simulink library "Orientation_Library"  (Simulink 8.0)
settings: Solver=ode1  StartTime=0.0  StopTime=inf  FixedStep=0.002  RelTol=1e-3
undefined symbols (not defined in the file or in its folder): qc_get_step_size
libraries: Orientation_Library x28, quarc_library x2, simulink x1
settings Model: Creator=glai  LastModifiedBy=glai  ExtModeTrigDuration=5000

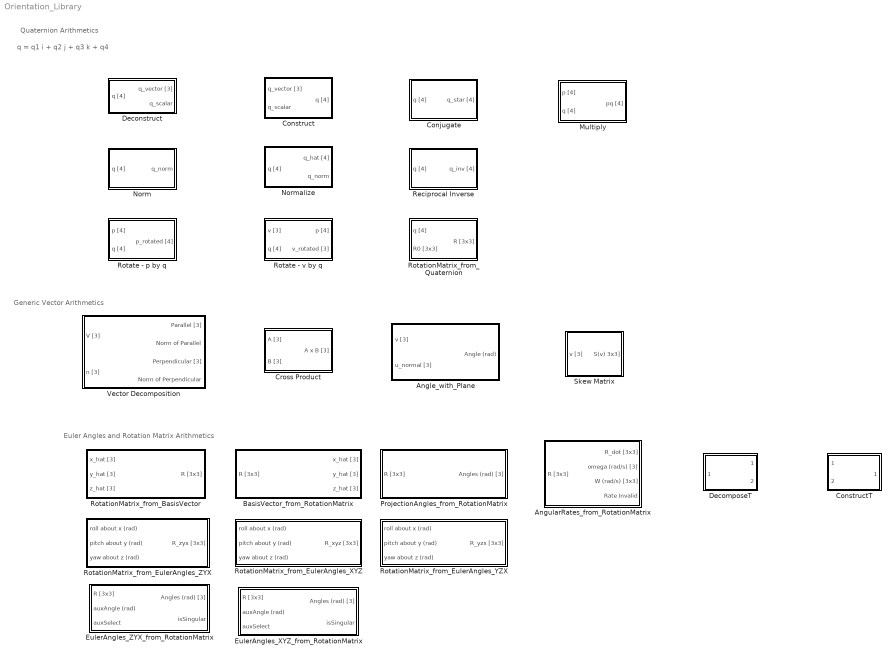
== system Orientation_Library ==
  note: Quaternion Arithmetics
  note: q = q1 i + q2 j + q3 k + q4
  note: Generic Vector Arithmetics
  note: Euler Angles and Rotation Matrix Arithmetics
  Angle_with_Plane : Subsystem
  AngularRates_from_RotationMatrix : Subsystem
  BasisVector_from_RotationMatrix : Subsystem
  Conjugate : Subsystem
  Construct : Subsystem
  ConstructT : Subsystem
  Cross Product : Subsystem
  DecomposeT : Subsystem
  Deconstruct : Subsystem
  EulerAngles_XYZ_from_RotationMatrix : Subsystem
  EulerAngles_ZYX_from_RotationMatrix : Subsystem
  Multiply : Subsystem
  Norm : Subsystem
  Normalize : Subsystem
  ProjectionAngles_from_RotationMatrix : Subsystem
  Reciprocal Inverse : Subsystem
  Rotate - p by q : Subsystem
  Rotate - v by q : Subsystem
  RotationMatrix_from_BasisVector : Subsystem
  RotationMatrix_from_EulerAngles_XYZ : Subsystem
  RotationMatrix_from_EulerAngles_YZX : Subsystem
  RotationMatrix_from_EulerAngles_ZYX : Subsystem
  RotationMatrix_from_Quaternion : Subsystem
  Skew Matrix : Subsystem
  Vector Decomposition : Subsystem

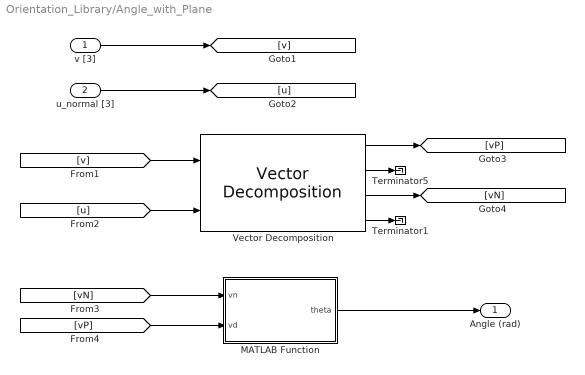
== system Orientation_Library/Angle_with_Plane ==
  v [3] : Inport
  u_normal [3] : Inport  Port=2
  MATLAB Function : MATLAB Function  TreatAsAtomicUnit=on
      settings: PermitHierarchicalResolution=ParametersOnly
  Terminator1 : Terminator
  Terminator5 : Terminator
  Vector Decomposition : Orientation_Library/Vector Decomposition
  Angle (rad) : Outport
  wires:
  v [3]/1 -> [v]
  u_normal [3]/1 -> [u]
  [v] -> Vector Decomposition/1
  [u] -> Vector Decomposition/2
  Vector Decomposition/1 -> [vP]
  Vector Decomposition/2 -> Terminator5/1
  Vector Decomposition/3 -> [vN]
  Vector Decomposition/4 -> Terminator1/1
  MATLAB Function/1(theta) -> Angle (rad)/1
  [vN] -> MATLAB Function/1(vn)
  [vP] -> MATLAB Function/2(vd)

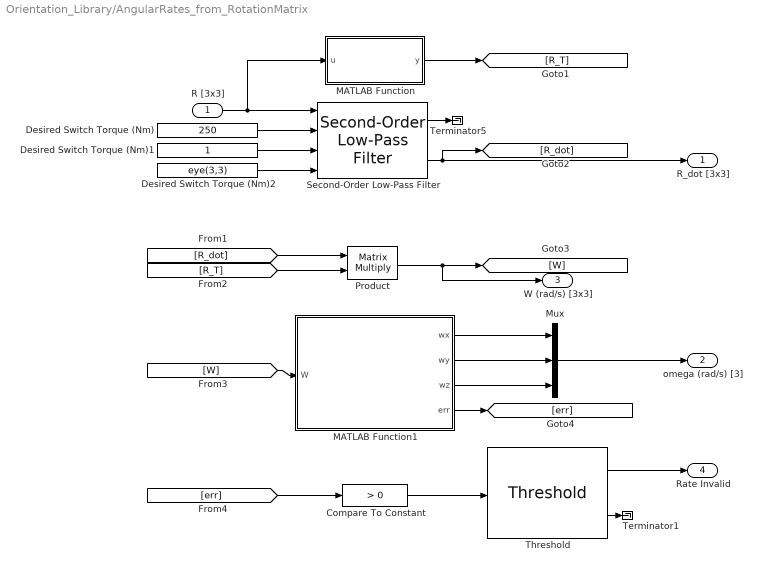
== system Orientation_Library/AngularRates_from_RotationMatrix ==
  R [3x3] : Inport
  Compare To Constant : simulink/Logic and Bit Operations/Compare To Constant  relop=>  const=0  OutDataTypeStr=uint8
  Desired Switch Torque (Nm) : Constant  Value=250
  Desired Switch Torque (Nm)1 : Constant
  Desired Switch Torque (Nm)2 : Constant  Value=eye(3,3)
  MATLAB Function : MATLAB Function  TreatAsAtomicUnit=on
      settings: PermitHierarchicalResolution=ParametersOnly
  MATLAB Function1 : MATLAB Function  TreatAsAtomicUnit=on
      settings: PermitHierarchicalResolution=ParametersOnly
  Mux : Mux  Inputs=3
  Product : Product  Multiplication=Matrix(*)  RndMeth=Zero
  Second-Order Low-Pass Filter : quarc_library/Continuous/Second-Order Low-Pass Filter  params_source=External (input ports)  input_width=1  input_zeta=1  input_init=0
  Terminator1 : Terminator
  Terminator5 : Terminator
  Threshold : quarc_library/Discontinuities/Threshold  operator=>  param_src=Specify via dialog  threshold=0  duration=qc_get_step_size*5000
  R_dot [3x3] : Outport
  omega (rad/s) [3] : Outport  Port=2
  W (rad/s) [3x3] : Outport  Port=3
  Rate Invalid : Outport  Port=4
  wires:
  Threshold/1 -> Rate Invalid/1
  Threshold/2 -> Terminator1/1
  Compare To Constant/1 -> Threshold/1
  Desired Switch Torque (Nm)2/1 -> Second-Order Low-Pass Filter/4
  Desired Switch Torque (Nm)1/1 -> Second-Order Low-Pass Filter/3
  Desired Switch Torque (Nm)/1 -> Second-Order Low-Pass Filter/2
  [err] -> Compare To Constant/1
  Mux/1 -> omega (rad/s) [3]/1
  MATLAB Function1/4(err) -> [err]
  MATLAB Function1/3(wz) -> Mux/3
  MATLAB Function1/2(wy) -> Mux/2
  MATLAB Function1/1(wx) -> Mux/1
  [W] -> MATLAB Function1/1(W)
  Product/1 -> W (rad/s) [3x3]/1, [W]
  [R_T] -> Product/2
  MATLAB Function/1(y) -> [R_T]
  [R_dot] -> Product/1
  Second-Order Low-Pass Filter/2 -> [R_dot], R_dot [3x3]/1
  Second-Order Low-Pass Filter/1 -> Terminator5/1
  R [3x3]/1 -> MATLAB Function/1(u), Second-Order Low-Pass Filter/1

== system Orientation_Library/BasisVector_from_RotationMatrix ==
  R [3x3] : Inport
  BasisVector_from_RotationMatrix : MATLAB Function  TreatAsAtomicUnit=on
      settings: PermitHierarchicalResolution=ParametersOnly
  x_hat [3] : Outport
  y_hat [3] : Outport  Port=2
  z_hat [3] : Outport  Port=3
  wires:
  R [3x3]/1 -> BasisVector_from_RotationMatrix/1(R)
  BasisVector_from_RotationMatrix/1(x_hat) -> x_hat [3]/1
  BasisVector_from_RotationMatrix/2(y_hat) -> y_hat [3]/1
  BasisVector_from_RotationMatrix/3(z_hat) -> z_hat [3]/1

== system Orientation_Library/Conjugate ==
  q [4] : Inport
  Demux : Demux  Outputs=[3 1]
  Gain : Gain  Gain=-1
  Mux : Mux  Inputs=[3 1]
  q_star [4] : Outport
  wires:
  Demux/1 -> Gain/1
  Gain/1 -> Mux/1
  Demux/2 -> Mux/2
  q [4]/1 -> Demux/1
  Mux/1 -> q_star [4]/1

== system Orientation_Library/Construct ==
  q_vector [3] : Inport
  q_scalar : Inport  Port=2
  Mux : Mux  Inputs=[3 1]
  q [4] : Outport
  wires:
  Mux/1 -> q [4]/1
  q_vector [3]/1 -> Mux/1
  q_scalar/1 -> Mux/2

== system Orientation_Library/ConstructT ==
  R [3x3] : Inport
  P (m) [3] : Inport  Port=2
  MATLAB Function3 : MATLAB Function  TreatAsAtomicUnit=on
      settings: PermitHierarchicalResolution=ParametersOnly
  T [4x4] : Outport
  wires:
  MATLAB Function3/1(T) -> T [4x4]/1
  P (m) [3]/1 -> MATLAB Function3/2(P)
  R [3x3]/1 -> MATLAB Function3/1(R)

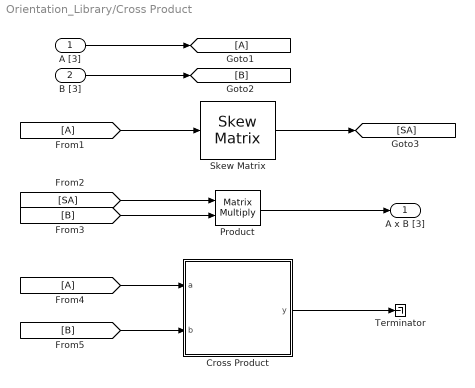
== system Orientation_Library/Cross Product ==
  A [3] : Inport
  B [3] : Inport  Port=2
  Cross Product : MATLAB Function  TreatAsAtomicUnit=on
      settings: PermitHierarchicalResolution=ParametersOnly
  Product : Product  Multiplication=Matrix(*)  RndMeth=Zero
  Skew Matrix : Orientation_Library/Skew Matrix
  Terminator : Terminator
  A x B [3] : Outport
  wires:
  B [3]/1 -> [B]
  A [3]/1 -> [A]
  [A] -> Skew Matrix/1
  Skew Matrix/1 -> [SA]
  [SA] -> Product/1
  [B] -> Product/2
  Product/1 -> A x B [3]/1
  [A] -> Cross Product/1(a)
  [B] -> Cross Product/2(b)
  Cross Product/1(y) -> Terminator/1

== system Orientation_Library/DecomposeT ==
  T [4x4] : Inport
  MATLAB Function1 : MATLAB Function  TreatAsAtomicUnit=on
      settings: PermitHierarchicalResolution=ParametersOnly
  R [3x3] : Outport
  P (m) [3] : Outport  Port=2
  wires:
  MATLAB Function1/2(P) -> P (m) [3]/1
  MATLAB Function1/1(R) -> R [3x3]/1
  T [4x4]/1 -> MATLAB Function1/1(T)

== system Orientation_Library/Deconstruct ==
  q [4] : Inport
  Demux : Demux  Outputs=[3 1]
  q_vector [3] : Outport
  q_scalar : Outport  Port=2
  wires:
  q [4]/1 -> Demux/1
  Demux/1 -> q_vector [3]/1
  Demux/2 -> q_scalar/1

== system Orientation_Library/EulerAngles_XYZ_from_RotationMatrix ==
  R [3x3] : Inport
  auxAngle (rad) : Inport  Port=2
  auxSelect : Inport  Port=3
  EulerAngles_xyz_from_RotationMatrix : MATLAB Function  TreatAsAtomicUnit=on
      settings: PermitHierarchicalResolution=ParametersOnly
  Angles (rad) [3] : Outport
  isSingular : Outport  Port=2
  wires:
  EulerAngles_xyz_from_RotationMatrix/1(Angles) -> Angles (rad) [3]/1
  EulerAngles_xyz_from_RotationMatrix/2(isSingular) -> isSingular/1
  R [3x3]/1 -> EulerAngles_xyz_from_RotationMatrix/1(R)
  auxAngle (rad)/1 -> EulerAngles_xyz_from_RotationMatrix/2(auxAngle)
  auxSelect/1 -> EulerAngles_xyz_from_RotationMatrix/3(auxSelect)

== system Orientation_Library/EulerAngles_ZYX_from_RotationMatrix ==
  R [3x3] : Inport
  auxAngle (rad) : Inport  Port=2
  auxSelect : Inport  Port=3
  EulerAngles_zyx_from_RotationMatrix : MATLAB Function  TreatAsAtomicUnit=on
      settings: PermitHierarchicalResolution=ParametersOnly
  Angles (rad) [3] : Outport
  isSingular : Outport  Port=2
  wires:
  EulerAngles_zyx_from_RotationMatrix/2(isSingular) -> isSingular/1
  EulerAngles_zyx_from_RotationMatrix/1(Angles) -> Angles (rad) [3]/1
  auxSelect/1 -> EulerAngles_zyx_from_RotationMatrix/3(auxSelect)
  auxAngle (rad)/1 -> EulerAngles_zyx_from_RotationMatrix/2(auxAngle)
  R [3x3]/1 -> EulerAngles_zyx_from_RotationMatrix/1(R)

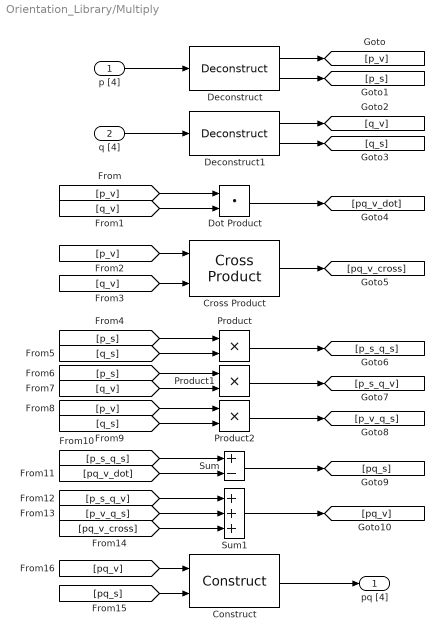
== system Orientation_Library/Multiply ==
  p [4] : Inport
  q [4] : Inport  Port=2
  Construct : Orientation_Library/Construct
  Cross Product : Orientation_Library/Cross Product
  Deconstruct : Orientation_Library/Deconstruct
  Deconstruct1 : Orientation_Library/Deconstruct
  Dot Product : DotProduct  InputSameDT=on  OutDataTypeStr=Inherit: Inherit via internal rule
  Product : Product  RndMeth=Zero
  Product1 : Product  RndMeth=Zero
  Product2 : Product  RndMeth=Zero
  Sum : Sum  Inputs=+-
  Sum1 : Sum  Inputs=+++
  pq [4] : Outport
  wires:
  p [4]/1 -> Deconstruct/1
  q [4]/1 -> Deconstruct1/1
  Deconstruct/1 -> [p_v]
  Deconstruct/2 -> [p_s]
  Deconstruct1/1 -> [q_v]
  Deconstruct1/2 -> [q_s]
  [p_v] -> Dot Product/1
  [q_v] -> Dot Product/2
  Dot Product/1 -> [pq_v_dot]
  [p_v] -> Cross Product/1
  [q_v] -> Cross Product/2
  Cross Product/1 -> [pq_v_cross]
  [p_s] -> Product/1
  [q_s] -> Product/2
  Product/1 -> [p_s_q_s]
  [p_s] -> Product1/1
  [q_v] -> Product1/2
  Product1/1 -> [p_s_q_v]
  [p_v] -> Product2/1
  [q_s] -> Product2/2
  Product2/1 -> [p_v_q_s]
  [p_s_q_s] -> Sum/1
  [pq_v_dot] -> Sum/2
  Sum/1 -> [pq_s]
  [p_s_q_v] -> Sum1/1
  [p_v_q_s] -> Sum1/2
  Sum1/1 -> [pq_v]
  [pq_v_cross] -> Sum1/3
  [pq_v] -> Construct/1
  [pq_s] -> Construct/2
  Construct/1 -> pq [4]/1

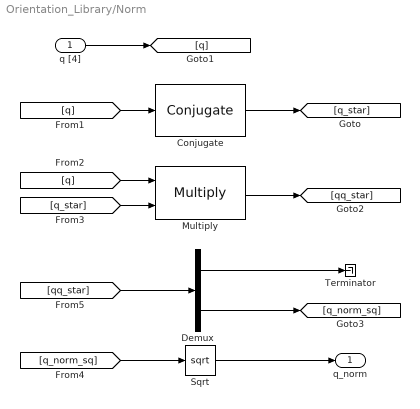
== system Orientation_Library/Norm ==
  q [4] : Inport
  Conjugate : Orientation_Library/Conjugate
  Demux : Demux  Outputs=[3 1]
  Multiply : Orientation_Library/Multiply
  Sqrt : Sqrt  SaturateOnIntegerOverflow=on
  Terminator : Terminator
  q_norm : Outport
  wires:
  Conjugate/1 -> [q_star]
  q [4]/1 -> [q]
  [q] -> Conjugate/1
  [q_norm_sq] -> Sqrt/1
  Sqrt/1 -> q_norm/1
  [q] -> Multiply/1
  [q_star] -> Multiply/2
  Multiply/1 -> [qq_star]
  [qq_star] -> Demux/1
  Demux/1 -> Terminator/1
  Demux/2 -> [q_norm_sq]

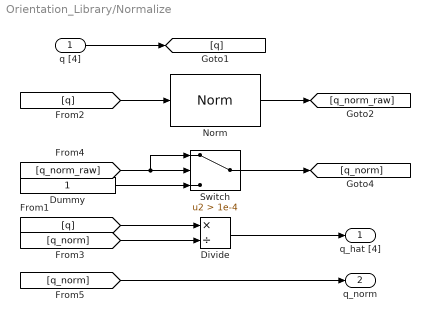
== system Orientation_Library/Normalize ==
  q [4] : Inport
  Divide : Product  Inputs=*/
  Dummy : Constant
  Norm : Orientation_Library/Norm
  Switch : Switch  Criteria=u2 > Threshold  Threshold=1e-4
  q_hat [4] : Outport
  q_norm : Outport  Port=2
  wires:
  q [4]/1 -> [q]
  Norm/1 -> [q_norm_raw]
  [q] -> Norm/1
  [q] -> Divide/1
  [q_norm] -> Divide/2
  [q_norm_raw] -> Switch/1, Switch/2
  Dummy/1 -> Switch/3
  Switch/1 -> [q_norm]
  Divide/1 -> q_hat [4]/1
  [q_norm] -> q_norm/1

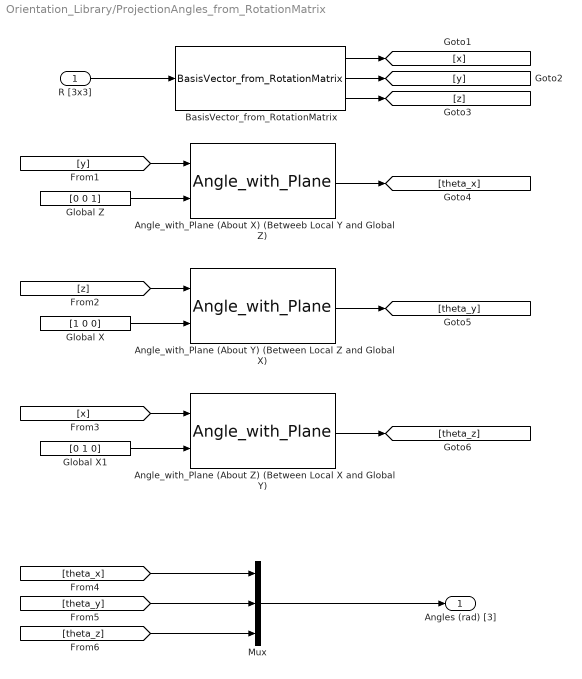
== system Orientation_Library/ProjectionAngles_from_RotationMatrix ==
  R [3x3] : Inport
  "Angle_with_Plane (About X) (Betweeb Local Y and Global Z) " : Orientation_Library/Angle_with_Plane
  Angle_with_Plane (About Y) (Between Local Z and Global X) : Orientation_Library/Angle_with_Plane
  Angle_with_Plane (About Z) (Between Local X and Global Y) : Orientation_Library/Angle_with_Plane
  BasisVector_from_RotationMatrix : Orientation_Library/BasisVector_from_RotationMatrix
  Global X : Constant  Value=[1 0 0]
  Global X1 : Constant  Value=[0 1 0]
  Global Z : Constant  Value=[0 0 1]
  Mux : Mux  Inputs=3
  Angles (rad) [3] : Outport
  wires:
  R [3x3]/1 -> BasisVector_from_RotationMatrix/1
  [y] -> "Angle_with_Plane (About X) (Betweeb Local Y and Global Z) "/1
  Global Z/1 -> "Angle_with_Plane (About X) (Betweeb Local Y and Global Z) "/2
  "Angle_with_Plane (About X) (Betweeb Local Y and Global Z) "/1 -> [theta_x]
  [z] -> Angle_with_Plane (About Y) (Between Local Z and Global X)/1
  Global X/1 -> Angle_with_Plane (About Y) (Between Local Z and Global X)/2
  Angle_with_Plane (About Y) (Between Local Z and Global X)/1 -> [theta_y]
  [x] -> Angle_with_Plane (About Z) (Between Local X and Global Y)/1
  Global X1/1 -> Angle_with_Plane (About Z) (Between Local X and Global Y)/2
  Angle_with_Plane (About Z) (Between Local X and Global Y)/1 -> [theta_z]
  Mux/1 -> Angles (rad) [3]/1
  [theta_x] -> Mux/1
  [theta_y] -> Mux/2
  [theta_z] -> Mux/3
  BasisVector_from_RotationMatrix/1 -> [x]
  BasisVector_from_RotationMatrix/2 -> [y]
  BasisVector_from_RotationMatrix/3 -> [z]

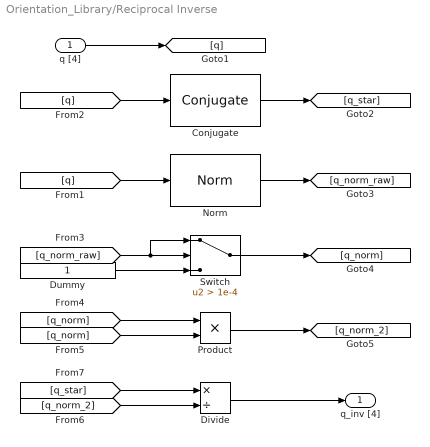
== system Orientation_Library/Reciprocal Inverse ==
  q [4] : Inport
  Conjugate : Orientation_Library/Conjugate
  Divide : Product  Inputs=*/
  Dummy : Constant
  Norm : Orientation_Library/Norm
  Product : Product  RndMeth=Zero
  Switch : Switch  Criteria=u2 > Threshold  Threshold=1e-4
  q_inv [4] : Outport
  wires:
  q [4]/1 -> [q]
  [q] -> Conjugate/1
  Conjugate/1 -> [q_star]
  [q] -> Norm/1
  Norm/1 -> [q_norm_raw]
  [q_norm_raw] -> Switch/1, Switch/2
  Dummy/1 -> Switch/3
  Switch/1 -> [q_norm]
  [q_norm] -> Product/1
  [q_norm] -> Product/2
  Product/1 -> [q_norm_2]
  [q_star] -> Divide/1
  [q_norm_2] -> Divide/2
  Divide/1 -> q_inv [4]/1

== system Orientation_Library/Rotate - p by q ==
  p [4] : Inport
  q [4] : Inport  Port=2
  Multiply : Orientation_Library/Multiply
  Multiply1 : Orientation_Library/Multiply
  Reciprocal Inverse : Orientation_Library/Reciprocal Inverse
  p_rotated [4] : Outport
  wires:
  Multiply/1 -> [qp]
  [p] -> Multiply/2
  [q] -> Multiply/1
  [q] -> Reciprocal Inverse/1
  p [4]/1 -> [p]
  Reciprocal Inverse/1 -> [q_inv]
  q [4]/1 -> [q]
  [qp] -> Multiply1/1
  [q_inv] -> Multiply1/2
  Multiply1/1 -> p_rotated [4]/1

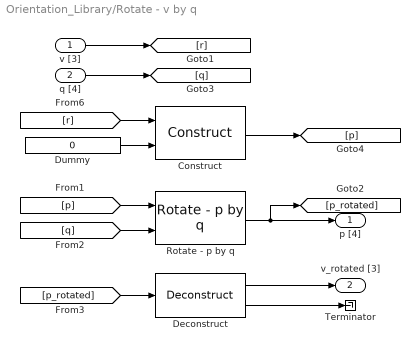
== system Orientation_Library/Rotate - v by q ==
  v [3] : Inport
  q [4] : Inport  Port=2
  Construct : Orientation_Library/Construct
  Deconstruct : Orientation_Library/Deconstruct
  Dummy : Constant  Value=0
  Rotate - p by q : Orientation_Library/Rotate - p by q
  Terminator : Terminator
  p [4] : Outport
  v_rotated [3] : Outport  Port=2
  wires:
  q [4]/1 -> [q]
  v [3]/1 -> [r]
  [r] -> Construct/1
  Dummy/1 -> Construct/2
  Construct/1 -> [p]
  [p] -> Rotate - p by q/1
  [q] -> Rotate - p by q/2
  Rotate - p by q/1 -> p [4]/1, [p_rotated]
  Deconstruct/1 -> v_rotated [3]/1
  [p_rotated] -> Deconstruct/1
  Deconstruct/2 -> Terminator/1

== system Orientation_Library/RotationMatrix_from_BasisVector ==
  x_hat [3] : Inport
  y_hat [3] : Inport  Port=2
  z_hat [3] : Inport  Port=3
  RotationMatrix_from_BasisVector : MATLAB Function  TreatAsAtomicUnit=on
      settings: PermitHierarchicalResolution=ParametersOnly
  R [3x3] : Outport
  wires:
  RotationMatrix_from_BasisVector/1(R) -> R [3x3]/1
  z_hat [3]/1 -> RotationMatrix_from_BasisVector/3(z_hat)
  y_hat [3]/1 -> RotationMatrix_from_BasisVector/2(y_hat)
  x_hat [3]/1 -> RotationMatrix_from_BasisVector/1(x_hat)

== system Orientation_Library/RotationMatrix_from_EulerAngles_XYZ ==
  roll about x (rad) : Inport
  pitch about y (rad) : Inport  Port=2
  yaw about z (rad) : Inport  Port=3
  RotationMatrix_from_EulerAngles_xyz : MATLAB Function  TreatAsAtomicUnit=on
      settings: PermitHierarchicalResolution=ParametersOnly
  R_xyz [3x3] : Outport
  wires:
  RotationMatrix_from_EulerAngles_xyz/1(R) -> R_xyz [3x3]/1
  yaw about z (rad)/1 -> RotationMatrix_from_EulerAngles_xyz/3(yaw)
  pitch about y (rad)/1 -> RotationMatrix_from_EulerAngles_xyz/2(pitch)
  roll about x (rad)/1 -> RotationMatrix_from_EulerAngles_xyz/1(roll)

== system Orientation_Library/RotationMatrix_from_EulerAngles_YZX ==
  roll about x (rad) : Inport
  pitch about y (rad) : Inport  Port=2
  yaw about z (rad) : Inport  Port=3
  RotationMatrix_from_EulerAngles_yzx : MATLAB Function  TreatAsAtomicUnit=on
      settings: PermitHierarchicalResolution=ParametersOnly
  R_yzx [3x3] : Outport
  wires:
  roll about x (rad)/1 -> RotationMatrix_from_EulerAngles_yzx/1(roll)
  pitch about y (rad)/1 -> RotationMatrix_from_EulerAngles_yzx/2(pitch)
  yaw about z (rad)/1 -> RotationMatrix_from_EulerAngles_yzx/3(yaw)
  RotationMatrix_from_EulerAngles_yzx/1(R) -> R_yzx [3x3]/1

== system Orientation_Library/RotationMatrix_from_EulerAngles_ZYX ==
  roll about x (rad) : Inport
  pitch about y (rad) : Inport  Port=2
  yaw about z (rad) : Inport  Port=3
  RotationMatrix_from_EulerAngles_zyx : MATLAB Function  TreatAsAtomicUnit=on
      settings: PermitHierarchicalResolution=ParametersOnly
  R_zyx [3x3] : Outport
  wires:
  RotationMatrix_from_EulerAngles_zyx/1(R) -> R_zyx [3x3]/1
  yaw about z (rad)/1 -> RotationMatrix_from_EulerAngles_zyx/3(yaw)
  pitch about y (rad)/1 -> RotationMatrix_from_EulerAngles_zyx/2(pitch)
  roll about x (rad)/1 -> RotationMatrix_from_EulerAngles_zyx/1(roll)

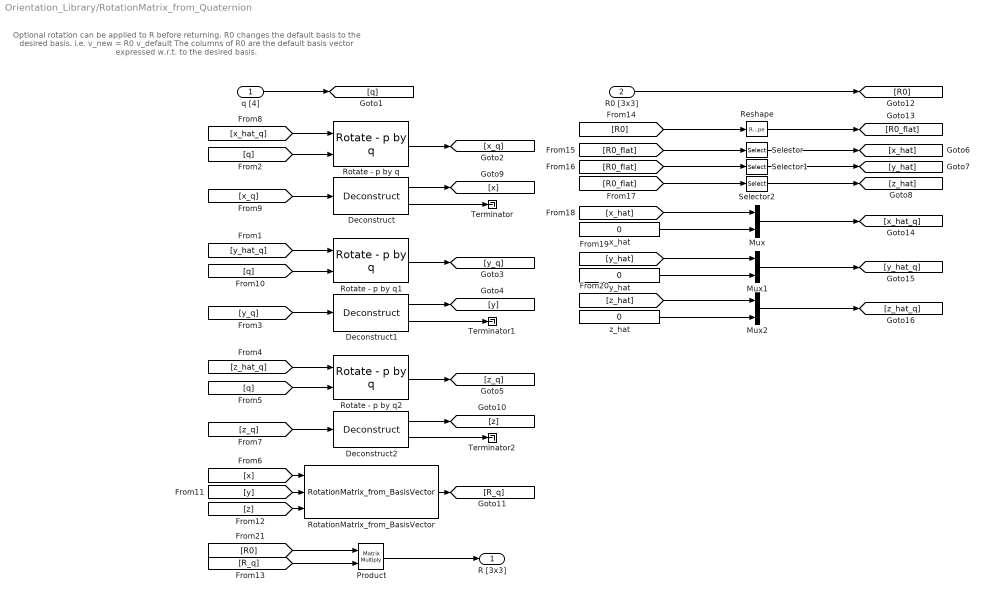
== system Orientation_Library/RotationMatrix_from_Quaternion ==
  note: Optional rotation can be applied to R before returning.
      | R0 changes the default basis to the desired basis.
      |
      | i.e. v_new = R0 v_default
      |
      | The columns of R0 are the default basis vector expressed w.r.t. to the desired basis.
  q [4] : Inport
  R0 [3x3] : Inport  Port=2
  Deconstruct : Orientation_Library/Deconstruct
  Deconstruct1 : Orientation_Library/Deconstruct
  Deconstruct2 : Orientation_Library/Deconstruct
  Mux : Mux  Inputs=[3 1]
  Mux1 : Mux  Inputs=[3 1]
  Mux2 : Mux  Inputs=[3 1]
  Product : Product  Multiplication=Matrix(*)  RndMeth=Zero
  Reshape : Reshape
  Rotate - p by q : Orientation_Library/Rotate - p by q
  Rotate - p by q1 : Orientation_Library/Rotate - p by q
  Rotate - p by q2 : Orientation_Library/Rotate - p by q
  RotationMatrix_from_BasisVector : Orientation_Library/RotationMatrix_from_BasisVector
  Selector : Selector  InputPortWidth=9  Indices=[1,4,7]
  Selector1 : Selector  InputPortWidth=9  Indices=[2,5,8]
  Selector2 : Selector  InputPortWidth=9  Indices=[3,6,9]
  Terminator : Terminator
  Terminator1 : Terminator
  Terminator2 : Terminator
  x_hat : Constant  Value=0
  y_hat : Constant  Value=0
  z_hat : Constant  Value=0
  R [3x3] : Outport
  wires:
  [q] -> Rotate - p by q/2
  q [4]/1 -> [q]
  [x_hat_q] -> Rotate - p by q/1
  Rotate - p by q/1 -> [x_q]
  [x_q] -> Deconstruct/1
  Deconstruct/1 -> [x]
  Deconstruct/2 -> Terminator/1
  [y_hat_q] -> Rotate - p by q1/1
  [q] -> Rotate - p by q1/2
  Rotate - p by q1/1 -> [y_q]
  [y_q] -> Deconstruct1/1
  Deconstruct1/1 -> [y]
  Deconstruct1/2 -> Terminator1/1
  [z_hat_q] -> Rotate - p by q2/1
  [q] -> Rotate - p by q2/2
  Rotate - p by q2/1 -> [z_q]
  [z_q] -> Deconstruct2/1
  Deconstruct2/1 -> [z]
  Deconstruct2/2 -> Terminator2/1
  [x] -> RotationMatrix_from_BasisVector/1
  [y] -> RotationMatrix_from_BasisVector/2
  [z] -> RotationMatrix_from_BasisVector/3
  RotationMatrix_from_BasisVector/1 -> [R_q]
  Product/1 -> R [3x3]/1
  R0 [3x3]/1 -> [R0]
  [R0] -> Reshape/1
  Reshape/1 -> [R0_flat]
  [R0_flat] -> Selector/1
  Selector/1 -> [x_hat]
  [R0_flat] -> Selector1/1
  [R0_flat] -> Selector2/1
  Selector1/1 -> [y_hat]
  Selector2/1 -> [z_hat]
  [x_hat] -> Mux/1
  x_hat/1 -> Mux/2
  Mux/1 -> [x_hat_q]
  Mux1/1 -> [y_hat_q]
  [y_hat] -> Mux1/1
  y_hat/1 -> Mux1/2
  Mux2/1 -> [z_hat_q]
  [z_hat] -> Mux2/1
  z_hat/1 -> Mux2/2
  [R0] -> Product/1
  [R_q] -> Product/2

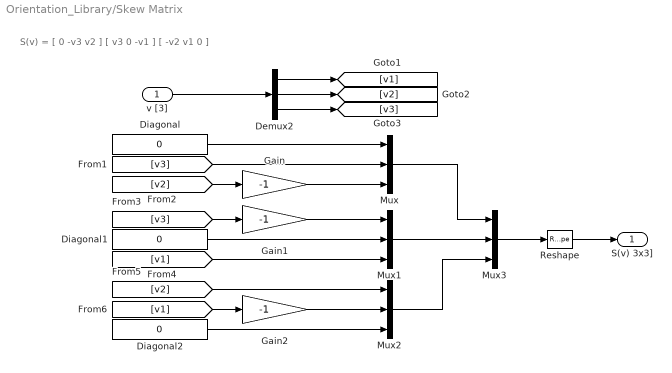
== system Orientation_Library/Skew Matrix ==
  note: S(v) = [ 0 -v3 v2 ]
      |           [ v3 0 -v1 ]
      |           [ -v2 v1 0 ]
  v [3] : Inport
  Demux2 : Demux  Outputs=3
  Diagonal : Constant  Value=0
  Diagonal1 : Constant  Value=0
  Diagonal2 : Constant  Value=0
  Gain : Gain  Gain=-1
  Gain1 : Gain  Gain=-1
  Gain2 : Gain  Gain=-1
  Mux : Mux  Inputs=3
  Mux1 : Mux  Inputs=3
  Mux2 : Mux  Inputs=3
  Mux3 : Mux  Inputs=[3 3 3]
  Reshape : Reshape  OutputDimensionality=Customize  OutputDimensions=[3,3]
  S(v) 3x3] : Outport
  wires:
  v [3]/1 -> Demux2/1
  Demux2/1 -> [v1]
  Demux2/2 -> [v2]
  Demux2/3 -> [v3]
  [v2] -> Gain/1
  Diagonal/1 -> Mux/1
  [v3] -> Mux/2
  Gain/1 -> Mux/3
  [v3] -> Gain1/1
  Gain1/1 -> Mux1/1
  Diagonal1/1 -> Mux1/2
  [v1] -> Mux1/3
  [v1] -> Gain2/1
  [v2] -> Mux2/1
  Gain2/1 -> Mux2/2
  Diagonal2/1 -> Mux2/3
  Mux/1 -> Mux3/1
  Mux1/1 -> Mux3/2
  Mux2/1 -> Mux3/3
  Mux3/1 -> Reshape/1
  Reshape/1 -> S(v) 3x3]/1

== system Orientation_Library/Vector Decomposition ==
  V [3] : Inport
  n [3] : Inport  Port=2
  Vector Decomposition : MATLAB Function  TreatAsAtomicUnit=on
      settings: PermitHierarchicalResolution=ParametersOnly
  Parallel [3] : Outport
  Norm of Parallel : Outport  Port=2
  Perpendicular [3] : Outport  Port=3
  Norm of Perpendicular : Outport  Port=4
  wires:
  Vector Decomposition/4(Perpendicular_norm) -> Norm of Perpendicular/1
  Vector Decomposition/2(Parallel_norm) -> Norm of Parallel/1
  Vector Decomposition/3(Perpendicular) -> Perpendicular [3]/1
  Vector Decomposition/1(Parallel) -> Parallel [3]/1
  n [3]/1 -> Vector Decomposition/2(n)
  V [3]/1 -> Vector Decomposition/1(V)

== matlab function RotationMatrix_from_EulerAngles_ZYX/RotationMatrix_from_EulerAngles_zyx ==
  data: roll input double; R output double; pitch input double; yaw input double
function R = RotationMatrix_from_EulerAngles_zyx(roll, pitch, yaw)
%#codegen

% Create rotation matrix from Euler (Z,Y,X) convention.

sRoll = sin(roll);
cRoll = cos(roll);
sPitch = sin(pitch);
cPitch = cos(pitch);
sYaw = sin(yaw);
cYaw =cos(yaw);

r11 = cPitch*cYaw;
r21 = cPitch*sYaw;
r31 = -sPitch;

r12 = sRoll*sPitch*cYaw - cRoll*sYaw;
r22 = sRoll*sPitch*sYaw + cRoll*cYaw;
r32 = sRoll*cPitch;

r13 = cRoll*sPitch*cYaw + sRoll*sYaw;
r23 = cRoll*sPitch*sYaw - sRoll*cYaw;
r33 = cRoll*cPitch;

R = [ r11, r12, r13; r21, r22, r23; r31, r32, r33 ];

== matlab function BasisVector_from_RotationMatrix/BasisVector_from_RotationMatrix ==
  data: R input double; x_hat output double; y_hat output double; z_hat output double
function [ x_hat, y_hat, z_hat ] = BasisVector_from_RotationMatrix(R)
%#codegen

x_hat = R(1:3,1);
y_hat = R(1:3,2);
z_hat = R(1:3,3);

== matlab function RotationMatrix_from_EulerAngles_XYZ/RotationMatrix_from_EulerAngles_xyz ==
  data: roll input double; R output double; pitch input double; yaw input double
function R = RotationMatrix_from_EulerAngles_xyz(roll, pitch, yaw)
%#codegen

% Create rotation matrix from Euler (X,Y,Z) convention.

sRoll = sin(roll);
cRoll = cos(roll);
sPitch = sin(pitch);
cPitch = cos(pitch);
sYaw = sin(yaw);
cYaw =cos(yaw);

r11 = cPitch*cYaw;
r21 = sRoll*sPitch*cYaw+cRoll*sYaw;
r31 = -cRoll*sPitch*cYaw+sRoll*sYaw;

r12 = -cPitch*sYaw;
r22 = -sRoll*sPitch*sYaw+cRoll*cYaw;
r32 = cRoll*sPitch*sYaw+sRoll*cPitch;

r13 = sPitch;
r23 = -sRoll*cPitch;
r33 = cRoll*cPitch;

R = [ r11, r12, r13; r21, r22, r23; r31, r32, r33 ];

== matlab function Angle_with_Plane/MATLAB Function ==
  data: vn input double; theta output double; vd input double
function theta = ComputeAngle(vn, vd)
%#codegen

n = norm(vn);
d = norm(vd);

if( d < eps )
    % Close to 90 deg
    theta = sign(vn) * pi/2;
else
    theta = atan2( n, d );
end;

== matlab function RotationMatrix_from_EulerAngles_YZX/RotationMatrix_from_EulerAngles_yzx ==
  data: roll input double; R output double; pitch input double; yaw input double
function R = RotationMatrix_from_EulerAngles_yzx(roll, pitch, yaw)
%#codegen

% Create rotation matrix from Euler (Y,Z, X) convention.

sRoll = sin(roll);
cRoll = cos(roll);
sPitch = sin(pitch);
cPitch = cos(pitch);
sYaw = sin(yaw);
cYaw =cos(yaw);

r11 = cPitch*cYaw;
r21 = sYaw;
r31 = -sPitch*cYaw;

r12 = -cPitch*sYaw*cRoll+sRoll*sPitch;
r22 = cRoll*cYaw;
r32 = cRoll*sPitch*sYaw+sRoll*cPitch;

r13 = cPitch*sYaw*sRoll+cRoll*sPitch;
r23 = -sRoll*cYaw;
r33 = -sRoll*sPitch*sYaw+cRoll*cPitch;

R = [ r11, r12, r13; r21, r22, r23; r31, r32, r33 ];

== matlab function Cross Product/Cross Product ==
  data: a input double; y output double; b input double
function y = CrossProduct(a,b)
%#codegen

y = [a(2)*b(3)-a(3)*b(2); a(3)*b(1)-a(1)*b(3); a(1)*b(2)-a(2)*b(1)];

== matlab function EulerAngles_XYZ_from_RotationMatrix/EulerAngles_xyz_from_RotationMatrix ==
  data: R input double; Angles output double; isSingular output double; auxAngle input double; auxSelect input double
function [Angles, isSingular]= EulerAngles_xyz_from_RotationMatrix(R, auxAngle, auxSelect)
%#codegen

% Extract the Euler angles (X-Y-Z) from rotatin matrix
% Assumption: 
% The rotation matrix is defined as:
%
% r0 = R . r1
%
% where r1 is a vector expressed in the rotated frame
%   r0 is the vector expressed in the reference frame

% Setting the singularity tolerance
tol = eps;

% Extract Euler angles from the rotation matrix
pitch = asin(R(1,3));
if( 1-abs(R(1,3)) > tol )
    % Not at Euler singularity
    isSingular = 0;
    roll = -atan2(R(2,3),R(3,3));
    yaw = -atan2(R(1,2),R(1,1));
else
    % At Euler singularity
    isSingular = 1;
    
    % Roll and Yaw are ambiguous.
    % Use the optional angular measurement to resolve the ambiguity
    RollYaw = acos(R(2,2));
    
    if( pitch > 0 )
        % pitch is +pi/2
        % RollYaw = Roll + Yaw
        % Therefore,
        % Roll = RollYaw - Yaw
        % Or 
        % Yaw = RollYaw - Roll
        if( auxSelect ~= 0 )    % Roll Aux measurement available
            roll = auxAngle;
            yaw = RollYaw - roll;
        else    % Yaw Aux measurement available
            yaw = auxAngle;
            roll = RollYaw - yaw;
        end
    else
        % pitch is -pi/2
        % RollYaw = Roll - Yaw
        % Therefore,
        % Roll = RollYaw + Yaw
        % Or
        % Yaw = -RollYaw + Roll
        if( auxSelect ~= 0 )    % Roll Aux measurement available
            roll = auxAngle;
            yaw = -RollYaw + roll;
        else    % Yaw Aux measurement available
            yaw = auxAngle;
            roll = RollYaw + yaw;
        end
    end
end

Angles = [ roll, pitch, yaw ]';

== matlab function Vector Decomposition/Vector Decomposition ==
  data: V input double; Parallel output double; Parallel_norm output double; Perpendicular output double; n input double; Perpendicular_norm output double
function [Parallel, Parallel_norm, Perpendicular, Perpendicular_norm]= VectorDecomposition(V, n)
%#codegen

% Decompose a vector into a parallel and perpendicular component
% along/about another vector. The magnitude (norm) of each of the
% components are also returned.
%
% Assumption: 
% n is the direction unit vector along with V is to be decomposed.
% V and n are expressed with respect to a consistent frame coordinate.

% Normalize n just in case
n_hat = n/norm(n);

Parallel_norm = dot(V, n_hat); 
Parallel = Parallel_norm*n_hat;

Perpendicular = V - Parallel;
Perpendicular_norm = norm( Perpendicular );

== matlab function DecomposeT/MATLAB Function1 ==
  data: R output double; P output double; T input double
function [R, P] = DecomposeT(T)
%#codegen

% Decompose Homogeneous Transformation Matrix into Rotation and Translation

R = T(1:3,1:3);
P = T(1:3,4);

== matlab function ConstructT/MATLAB Function3 ==
  data: R input double; P input double; T output double
function T = constructT(R, P)
%#codegen

% Construct Homegeneous Transformation Matrix from Rotation and Translation

T = [ R, P; zeros(1,3), 1];

== matlab function AngularRates_from_RotationMatrix/MATLAB Function ==
  data: u input double; y output double
function y = MatrixTranspose(u)
%#codegen

y = u';

== matlab function AngularRates_from_RotationMatrix/MATLAB Function1 ==
  data: W input double; wx output double; wy output double; wz output double; err output double
function [wx, wy, wz, err]= ExtractAngularRateVector(W)
%#codegen

% Extract the angular rate vector from the skew symmetric matrix
%
% W = [   0, -wz,  wy ]
%     [  wz,   0, -wx ]
%     [ -wy,  wx,   0 ]

% Checking the diagonal entry to be zero.
% Flag the err signal if it is not.
if( norm(diag(W)) > 0.1 )
    err = 1;
else
    err = 0;
end

wx = W(3,2);
wy = W(1,3);
wz = W(2,1);

== matlab function EulerAngles_ZYX_from_RotationMatrix/EulerAngles_zyx_from_RotationMatrix ==
  data: R input double; Angles output double; isSingular output double; auxAngle input double; auxSelect input double
function [Angles, isSingular]= EulerAngles_zyx_from_RotationMatrix(R, auxAngle, auxSelect)
%#codegen

% Extract the Euler angles (Z-Y-X) from rotatin matrix
% Assumption: 
% The rotation matrix is defined as:
%
% r0 = R . r1
%
% where r1 is a vector expressed in the rotated frame
%   r0 is the vector expressed in the reference frame

% Setting the singularity tolerance
tol = eps;

% Extract Euler angles from the rotation matrix
pitch = -asin(R(3,1));
if( 1-abs(R(3,1)) > tol )
    % Not at Euler singularity
    isSingular = 0;
    roll = atan2(R(3,2),R(3,3));
    yaw = atan2(R(2,1),R(1,1));
else
    % At Euler singularity
    isSingular = 1;
    
    % Roll and Yaw are ambiguous.
    % Use the optional angular measurement to resolve the ambiguity
    RollYaw = acos(R(2,2));
    
    if( pitch > 0 )
        % pitch is +pi/2
        % RollYaw = Roll + Yaw
        % Therefore,
        % Roll = RollYaw - Yaw
        % Or 
        % Yaw = RollYaw - Roll
        if( auxSelect ~= 0 )    % Roll Aux measurement available
            roll = auxAngle;
            yaw = RollYaw - roll;
        else    % Yaw Aux measurement available
            yaw = auxAngle;
            roll = RollYaw - yaw;
        end
    else
        % pitch is -pi/2
        % RollYaw = Roll - Yaw
        % Therefore,
        % Roll = RollYaw + Yaw
        % Or
        % Yaw = -RollYaw + Roll
        if( auxSelect ~= 0 )    % Roll Aux measurement available
            roll = auxAngle;
            yaw = -RollYaw + roll;
        else    % Yaw Aux measurement available
            yaw = auxAngle;
            roll = RollYaw + yaw;
        end
    end
end

Angles = [ roll, pitch, yaw ]';

== matlab function RotationMatrix_from_BasisVector/RotationMatrix_from_BasisVector ==
  data: x_hat input double; R output double; y_hat input double; z_hat input double
function R = RotationMatrix_fromBasis(x_hat, y_hat, z_hat)
%#codegen

% Construction the rotation matrix from the basis vectors
% Assumption: The basis vectors are expressed w.r.t. to the reference
% frame.
% The resulting rotation matrix is defined as:
%
% r0 = R . r1
%
% where r1 is a vector expressed in the rotated frame
%   r0 is the vector expressed in the reference frame


R = [x_hat, y_hat, z_hat];
